simulink model "nelinearnilqr"  (R2020b)
settings: Solver=VariableStepAuto  StartTime=0.0  StopTime=10.0  RelTol=1e-3
values from neighbouring files (symbols this model uses):
  b1 = 0.0050134512    [I_PD.m]    (also in LQR.m = 0.05; PODACI.m = 0.05; Untitled2.m)
  b2 = 45    [LQR.m]    (also in PODACI.m)
  c = 0.03    [LQR.m]    (also in PODACI.m)
  d = 0.062    [LQR.m]    (also in PODACI.m)
  g = 9.81    [LQR.m]    (also in PODACI.m)
  K = lqr(A,B,Q,R)    [LQR.m]
  m = 0.3    [LQR.m]    (also in PODACI.m)
  M = 1.2    [LQR.m]    (also in PODACI.m)
settings Model: Creator=Toni  LastModifiedBy=Toni

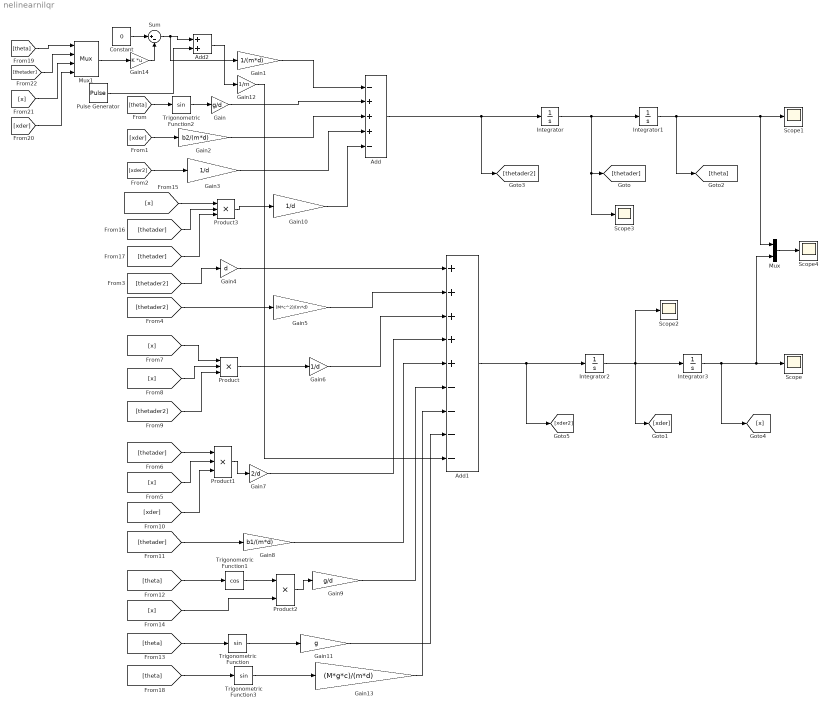
== system nelinearnilqr ==
  Add : Sum  Inputs=-+++-
  Add1 : Sum  Inputs=+++++----
  Add2 : Sum
  Constant : Constant  Value=0
  Gain : Gain  Gain=g/d
  Gain1 : Gain  Gain=1/(m*d)
  Gain10 : Gain  Gain=1/d
  Gain11 : Gain  Gain=g
  Gain12 : Gain  Gain=1/m
  Gain13 : Gain  Gain=(M*g*c)/(m*d)
  Gain14 : Gain  Gain=K  Multiplication=Matrix(K*u)
  Gain2 : Gain  Gain=b2/(m*d)
  Gain3 : Gain  Gain=1/d
  Gain4 : Gain  Gain=d
  Gain5 : Gain  Gain=(M*c^2)/(m*d)
  Gain6 : Gain  Gain=1/d
  Gain7 : Gain  Gain=2/d
  Gain8 : Gain  Gain=b1/(m*d)
  Gain9 : Gain  Gain=g/d
  Integrator{,1..3} (4 alike) : Integrator
  Mux : Mux  Inputs=2
  Mux1 : Mux
  Product{,1..3} (4 alike) : Product  Inputs=3
  Pulse Generator : DiscretePulseGenerator  PulseType=Time based  Period=10  PulseWidth=5
  Scope{,1..4} (5 alike) : Scope
  Sum : Sum  Inputs=|+-
  Trigonometric Function : Trigonometry
  Trigonometric Function1 : Trigonometry  Operator=cos
  Trigonometric Function2 : Trigonometry
  Trigonometric Function3 : Trigonometry
  wires:
  Gain13/1 -> Add1/7
  Trigonometric Function3/1 -> Gain13/1
  [x] -> Product3/1
  Gain10/1 -> Add/5
  [theta] -> Trigonometric Function2/1
  Product3/1 -> Gain10/1
  Trigonometric Function/1 -> Gain11/1
  Gain12/1 -> Add1/9
  Gain2/1 -> Add/3
  [xder] -> Gain2/1
  Integrator1/1 -> [theta], Mux/1, Scope1/1
  Add1/1 -> [xder2], Integrator2/1
  Product/1 -> Gain6/1
  [x] -> Product2/3
  [theta] -> Trigonometric Function/1
  Gain11/1 -> Add1/8
  Gain8/1 -> Add1/5
  Product2/1 -> Gain9/1
  Product1/1 -> Gain7/1
  [thetader] -> Gain8/1
  [xder] -> Product1/3
  [thetader2] -> Product/3
  Trigonometric Function1/1 -> Product2/1
  [thetader] -> Product1/1
  Trigonometric Function2/1 -> Gain/1
  Gain6/1 -> Add1/3
  [thetader] -> Product3/2
  [xder2] -> Gain3/1
  [theta] -> Trigonometric Function1/1
  [theta] -> Trigonometric Function3/1
  Gain5/1 -> Add1/2
  Gain4/1 -> Add1/1
  [x] -> Product1/2
  Gain1/1 -> Add/1
  [thetader2] -> Gain4/1
  [x] -> Product/1
  Integrator3/1 -> Mux/2, Scope/1, [x]
  Integrator2/1 -> Scope2/1, [xder], Integrator3/1
  Gain/1 -> Add/2
  Integrator/1 -> Scope3/1, [thetader], Integrator1/1
  Gain7/1 -> Add1/4
  Mux/1 -> Scope4/1
  Add/1 -> [thetader2], Integrator/1
  Gain3/1 -> Add/4
  [x] -> Product/2
  Gain9/1 -> Add1/6
  [thetader] -> Product3/3
  [thetader2] -> Gain5/1
  [theta] -> Mux1/1
  [thetader] -> Mux1/2
  [x] -> Mux1/3
  [xder] -> Mux1/4
  Constant/1 -> Sum/1
  Mux1/1 -> Gain14/1
  Sum/1 -> Gain1/1, Add2/1
  Gain14/1 -> Sum/2
  Pulse Generator/1 -> Add2/2
  Add2/1 -> Gain12/1
